simulink model "simulink_model_continuous"  (R2024a)
settings: Solver=VariableStepAuto  StartTime=0.0  StopTime=2  RelTol=1e-3
settings Model: Creator=hp  LastModifiedBy=hp

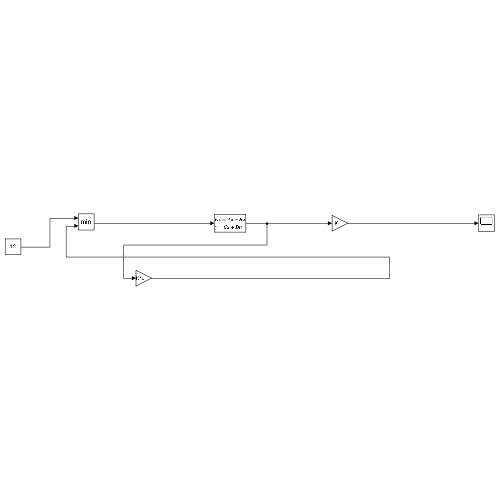
[thumbnail: Simulink's stored preview of the top-level diagram]
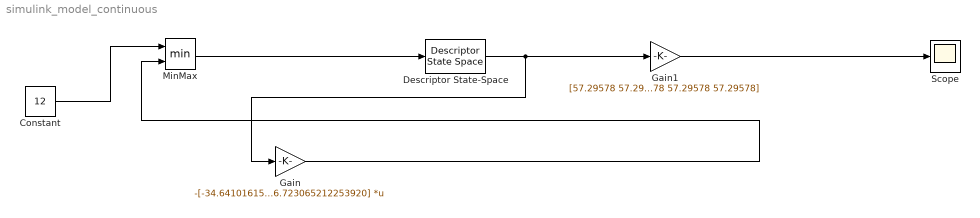
== system simulink_model_continuous ==
  Constant : Constant  Value=12
  Descriptor State-Space : DescriptorStateSpace  E=eye(4)  A=[[0, 0, 1, 0]; [0, 0, 0, 1]; [0, 123.9792, -1.5772, 0]; [0, 111.6234, -0.7253, 0]]  B=[0;0;56.389321700745840;25.930031257382012]  C=[[1 0 0 0]; [0 1 0 0]; [0 0 1 0]; [0 0 0 1]]  D=[0;0;0;0]  InitialCondition=[0.25; 0.035; 0; 0]
  Gain : Gain  Gain=-[-34.641016151376206,3.424425469457670e+02,-14.767527570011810,46.723065212253920]  Multiplication=Matrix(K*u)
  Gain1 : Gain  Gain=[57.29578 57.29578 57.29578 57.29578]
  MinMax : MinMax  Inputs=2  OutMin=2.4  OutMax=12
  Scope : Scope
  wires:
  Descriptor State-Space/1 -> Gain1/1, Gain/1
  Gain/1 -> MinMax/2
  Constant/1 -> MinMax/1
  MinMax/1 -> Descriptor State-Space/1
  Gain1/1 -> Scope/1
